simulink model "feedback_control_sine"  (R2021b)
settings: Solver=VariableStepAuto  StartTime=0.0  StopTime=20  RelTol=1e-3
undefined symbols (not defined in the file): Ts
libraries: cstblocks x1
settings Model: Creator=varunsampat  LastModifiedBy=varunsampat

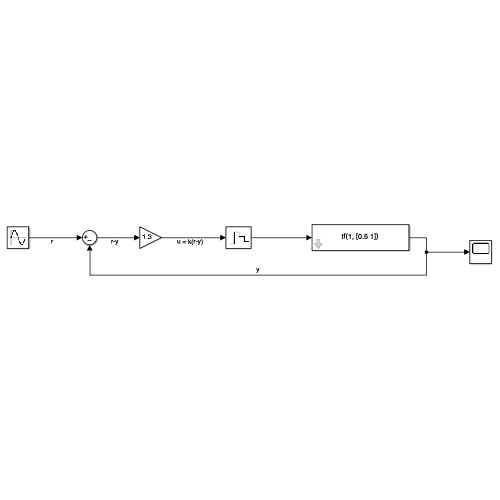
[thumbnail: Simulink's stored preview of the top-level diagram]
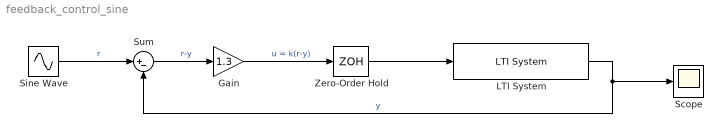
== system feedback_control_sine ==
  Gain : Gain  Gain=1.3
  LTI System : cstblocks/LTI System  sys=tf(1, [0.5 1])  IC=[]
  Scope : Scope
  Sine Wave : Sin  SampleTime=0
  Sum : Sum  Inputs=|+-
  Zero-Order Hold : ZeroOrderHold  SampleTime=Ts
  wires:
  Sum/1 -> Gain/1  "r-y"
  Sine Wave/1 -> Sum/1  "r"
  LTI System/1 -> Sum/2, Scope/1  "y"
  Gain/1 -> Zero-Order Hold/1  "u = k(r-y)"
  Zero-Order Hold/1 -> LTI System/1
